simulink model "q12b"  (R2024a)
settings: Solver=VariableStepAuto  StartTime=0.0  StopTime=10.0  RelTol=1e-3
settings Model: Creator=SHINE MOHAN S  LastModifiedBy=SHINE MOHAN S

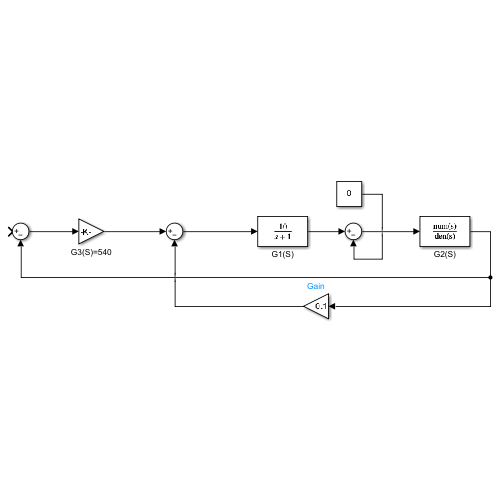
[thumbnail: Simulink's stored preview of the top-level diagram]
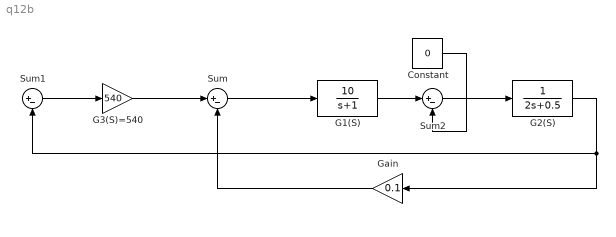
== system q12b ==
  Constant : Constant  Value=0
  G1(S) : TransferFcn  Numerator=[10]  Denominator=[1 1]
  G2(S) : TransferFcn  Denominator=[2 0.5]
  G3(S)=540 : Gain  Gain=540
  Gain : Gain  Gain=0.1
  Sum : Sum  Inputs=|+-
  Sum1 : Sum  Inputs=|+-
  Sum2 : Sum  Inputs=|+-
  wires:
  G2(S)/1 -> Sum1/2, Gain/1
  Sum1/1 -> G3(S)=540/1
  G3(S)=540/1 -> Sum/1
  Sum/1 -> G1(S)/1
  G1(S)/1 -> Sum2/1
  Sum2/1 -> G2(S)/1
  Constant/1 -> Sum2/2
  Gain/1 -> Sum/2
